simulink model "Model"  (R2016b)
settings: Solver=ode45  StartTime=0.0  StopTime=100  RelTol=1e-3
values from neighbouring files (symbols this model uses):
  b = 0.1    [main.m]
  g = 9.81    [main.m]
  H = [1 0 0 0 ... (first row only)    [main.m]
  K = lqr(A, B, Q, R )    [main.m]
  k = 0.15    [main.m]
  L = L_vec(i)    [main.m]
  M = 1    [main.m]
  m = 3/4    (= 0.75)    [main.m]
  Q = diag([1,1,1,1])    [main.m]
  R = 1    [main.m]
  theta_0 = 0    [main.m]
  theta_dot0 = 0    [main.m]
  x_0 = 0    [main.m]
  x_dot0 = 0    [main.m]
undefined symbols (not defined in the file or in its folder): delta, gamma, P_0, phi, X_0, y_0
libraries: simulink x3
settings Model: Creator=Erik  LastModifiedBy=sbuadu
settings DataIOCC: LimitDataPoints=on  SaveFormat=Array
settings OptimizationCC: BlockReduction=off  BooleanDataType=off  LifeSpan=inf
settings DebuggingCC: SaveWithParameterizedLinksMsg=none  UnderspecifiedInitializationDetection=Classic  MergeDetectMultiDrivingBlocksExec=none  SignalResolutionControl=TryResolveAllWithWarning  SFUnexpectedBacktrackingDiag=warning  SFNoUnconditionalDefaultTransitionDiag=warning  SFExecutionAtInitializationDiag=none
settings HardwareCC: ProdBitPerPointer=32  ProdBitPerSizeT=32  ProdBitPerPtrDiffT=32  ProdLargestAtomicFloat=None  ProdIntDivRoundTo=Undefined  ProdEndianess=Unspecified  ProdWordSize=32  ProdHWDeviceType=32-bit Generic  TargetUnknown=on
settings ModelReferenceCC: PropagateSignalLabelsOutOfModel=off
settings GRTTargetCC: TargetLangStandard=C89/C90 (ANSI)  GeneratePreprocessorConditionals=Disable all
settings ConfigComp: CovMetricSettings=dw  CovHtmlReporting=on  CovSaveCumulativeToWorkspaceVar=on  CovSaveSingleToWorkspaceVar=on  CovExternalEMLEnable=off  CovSFcnEnable=off

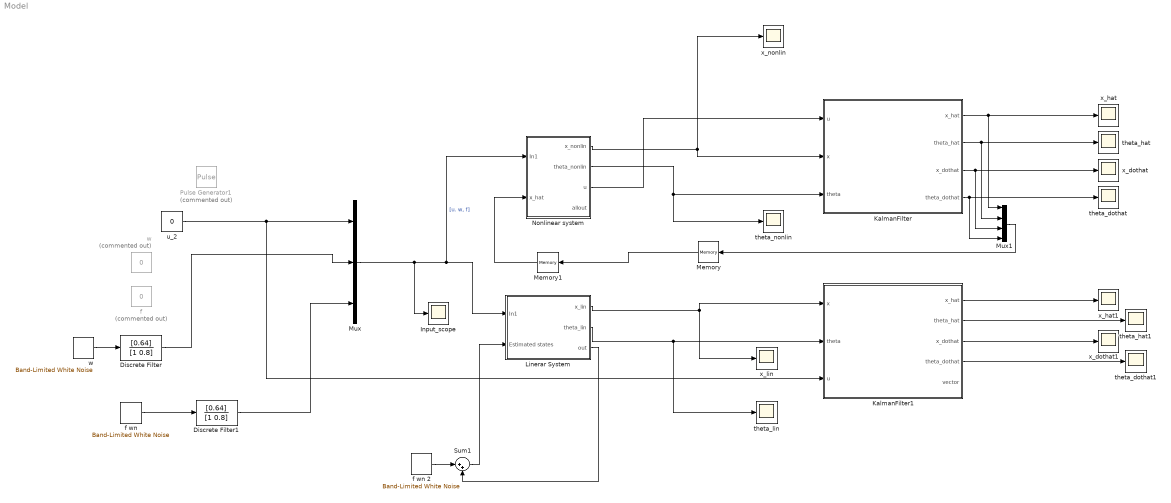
== system Model ==
  Discrete Filter : DiscreteFilter  Numerator=[0.64]  Denominator=[1 0.8]
  Discrete Filter1 : DiscreteFilter  Numerator=[0.64]  Denominator=[1 0.8]
  Input_scope : Scope
  KalmanFilter : Subsystem
  KalmanFilter1 : Subsystem
  Linerar System : Subsystem
  Memory : Memory  X0=X_0
  Memory1 : Memory  X0=X_0
  Mux : Mux  Inputs=3
  Mux1 : Mux
  "Nonlinear system " : Subsystem
  Pulse Generator1 : DiscretePulseGenerator  Commented=on  PulseType=Time based  Period=100  PhaseDelay=3
  Sum1 : Sum  Inputs=|++
  f : Constant  Commented=on  Value=0  SampleTime=0.01
  "f wn " : simulink/Sources/Band-Limited White Noise  Cov=10e-4  Ts=.001  seed=[23341]
  f wn 2 : simulink/Sources/Band-Limited White Noise  Cov=10e-7  Ts=.001  seed=[23341]
  theta_dothat : Scope
  theta_dothat1 : Scope
  theta_hat : Scope
  theta_hat1 : Scope
  theta_lin : Scope
  "theta_nonlin " : Scope
  u_2 : Constant  Value=0  SampleTime=0.01
  w : Constant  Commented=on  Value=0  SampleTime=0.01
  "w " : simulink/Sources/Band-Limited White Noise  Cov=10  Ts=.001  seed=[23341]
  x_dothat : Scope
  x_dothat1 : Scope
  x_hat : Scope
  x_hat1 : Scope
  x_lin : Scope
  x_nonlin : Scope
  wires:
  Mux/1 -> Input_scope/1, Linerar System/1(In1), "Nonlinear system "/1(In1)  "[u. w, f]"
  "Nonlinear system "/1(x_nonlin) -> KalmanFilter/2(x), x_nonlin/1
  "Nonlinear system "/2(theta_nonlin) -> KalmanFilter/3(theta), "theta_nonlin "/1
  u_2/1 -> KalmanFilter1/3("u "), Mux/1
  Linerar System/1(x_lin) -> KalmanFilter1/1(x), x_lin/1
  Linerar System/2(theta_lin) -> theta_lin/1, KalmanFilter1/2(theta)
  KalmanFilter/1(x_hat) -> Mux1/1, x_hat/1
  KalmanFilter/2(theta_hat) -> Mux1/2, theta_hat/1
  KalmanFilter/4(theta_dothat) -> Mux1/4, theta_dothat/1
  KalmanFilter1/1(x_hat) -> x_hat1/1
  KalmanFilter1/2(theta_hat) -> theta_hat1/1
  KalmanFilter1/3(x_dothat) -> x_dothat1/1
  KalmanFilter1/4(theta_dothat) -> theta_dothat1/1
  Mux1/1 -> Memory/1
  KalmanFilter/3(x_dothat) -> Mux1/3, x_dothat/1
  "Nonlinear system "/3(u) -> KalmanFilter/1("u ")
  Memory/1 -> Memory1/1
  Discrete Filter1/1 -> Mux/3
  "w "/1 -> Discrete Filter/1
  "f wn "/1 -> Discrete Filter1/1
  Discrete Filter/1 -> Mux/2
  Memory1/1 -> "Nonlinear system "/2(x_hat)
  Sum1/1 -> Linerar System/2(Estimated states)
  f wn 2/1 -> Sum1/1
  Linerar System/3("out ") -> Sum1/2

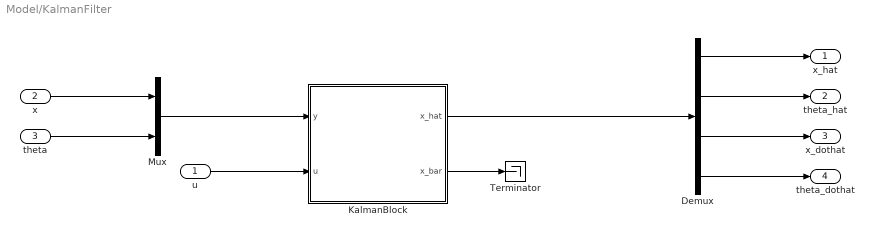
== system Model/KalmanFilter ==
  "u " : Inport
  x : Inport  Port=2
  theta : Inport  Port=3
  Demux : Demux
  KalmanBlock : Subsystem
  Mux : Mux  Inputs=2
  Terminator : Terminator
  x_hat : Outport
  theta_hat : Outport  Port=2
  x_dothat : Outport  Port=3
  theta_dothat : Outport  Port=4
  wires:
  Mux/1 -> KalmanBlock/1("y ")
  "u "/1 -> KalmanBlock/2("u ")
  x/1 -> Mux/1
  theta/1 -> Mux/2
  KalmanBlock/1(x_hat) -> Demux/1
  Demux/1 -> x_hat/1
  Demux/2 -> theta_hat/1
  Demux/3 -> x_dothat/1
  Demux/4 -> theta_dothat/1
  KalmanBlock/2(x_bar) -> Terminator/1

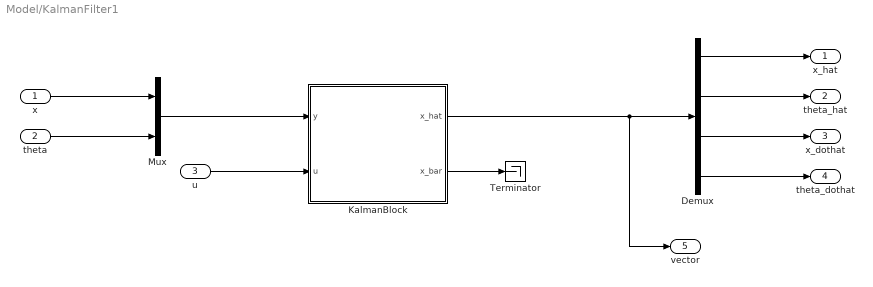
== system Model/KalmanFilter1 ==
  x : Inport
  theta : Inport  Port=2
  "u " : Inport  Port=3
  Demux : Demux
  KalmanBlock : Subsystem
  Mux : Mux  Inputs=2
  Terminator : Terminator
  x_hat : Outport
  theta_hat : Outport  Port=2
  x_dothat : Outport  Port=3
  theta_dothat : Outport  Port=4
  vector : Outport  Port=5
  wires:
  Mux/1 -> KalmanBlock/1("y ")
  "u "/1 -> KalmanBlock/2("u ")
  x/1 -> Mux/1
  theta/1 -> Mux/2
  KalmanBlock/1(x_hat) -> vector/1, Demux/1
  Demux/1 -> x_hat/1
  Demux/2 -> theta_hat/1
  Demux/3 -> x_dothat/1
  Demux/4 -> theta_dothat/1
  KalmanBlock/2(x_bar) -> Terminator/1

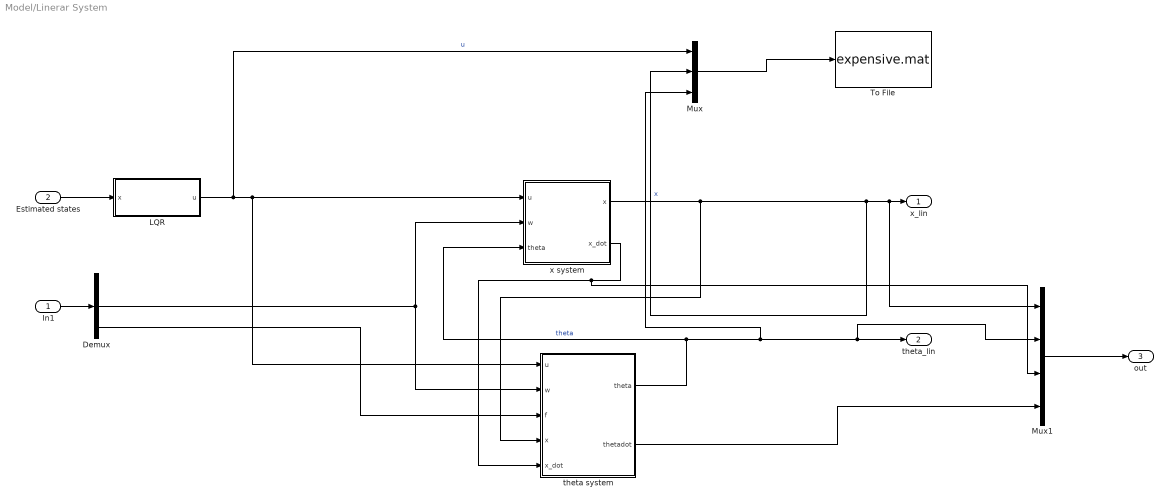
== system Model/Linerar System ==
  In1 : Inport
  Estimated states : Inport  Port=2
  Demux : Demux  Outputs=3
  LQR : Subsystem
  Mux : Mux  Inputs=3
  Mux1 : Mux
  To File : ToFile  Filename=expensive.mat  MatrixName=data
  "theta system " : Subsystem
  x system : Subsystem
  x_lin : Outport
  theta_lin : Outport  Port=2
  "out " : Outport  Port=3
  wires:
  Demux/2 -> "theta system "/2(w), x system/2(w)
  Demux/3 -> "theta system "/3(f)
  x system/2(x_dot) -> Mux1/3, "theta system "/5(x_dot)
  In1/1 -> Demux/1
  Estimated states/1 -> LQR/1(x)
  LQR/1(u) -> Mux/1, "theta system "/1("u "), x system/1("u ")  "u"
  x system/1(x) -> "theta system "/4(x), Mux/2, Mux1/1, x_lin/1  "x"
  "theta system "/1(theta) -> Mux/3, Mux1/2, theta_lin/1, x system/3(theta)  "theta"
  Mux/1 -> To File/1
  "theta system "/2("thetadot ") -> Mux1/4
  Mux1/1 -> "out "/1

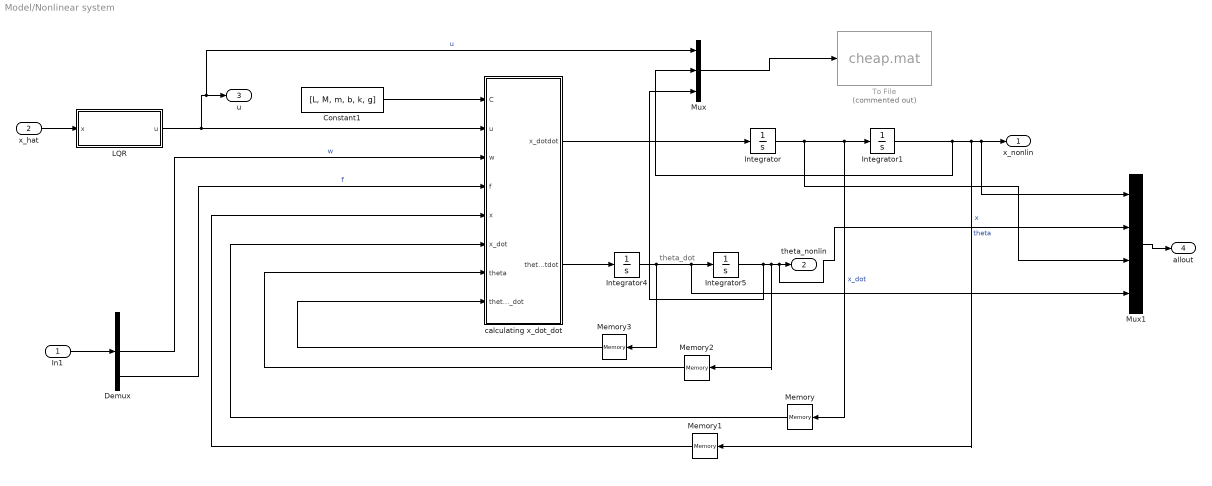
== system Model/Nonlinear system  ==
  note: theta_dot
  In1 : Inport
  x_hat : Inport  Port=2
  Constant1 : Constant  Value=[L, M, m, b, k, g]  SampleTime=0.01
  Demux : Demux  Outputs=3
  Integrator{,1,4..5} (4 alike) : Integrator
  LQR : Subsystem
  Memory : Memory  X0=x_dot0
  Memory1 : Memory  X0=x_0
  Memory2 : Memory  X0=theta_0
  Memory3 : Memory  X0=theta_dot0
  Mux : Mux  Inputs=3
  Mux1 : Mux
  To File : ToFile  Commented=on  Filename=cheap.mat  MatrixName=data
  calculating x_dot_dot : MATLAB Function  TreatAsAtomicUnit=on
  x_nonlin : Outport
  theta_nonlin : Outport  Port=2
  u : Outport  Port=3
  "allout " : Outport  Port=4
  wires:
  In1/1 -> Demux/1
  LQR/1(u) -> Mux/1, u/1, calculating x_dot_dot/2(u)  "u"
  Demux/2 -> calculating x_dot_dot/3(w)  "w"
  Demux/3 -> calculating x_dot_dot/4(f)  "f"
  calculating x_dot_dot/1(x_dotdot) -> Integrator/1
  Integrator/1 -> Mux1/3, Memory/1, Integrator1/1  "x_dot"
  Integrator1/1 -> Mux/2, Memory1/1, Mux1/1, x_nonlin/1  "x"
  Constant1/1 -> calculating x_dot_dot/1(C)
  calculating x_dot_dot/2(theta_dotdot) -> Integrator4/1
  Integrator4/1 -> Memory3/1, Mux1/4, Integrator5/1
  Integrator5/1 -> Mux/3, Memory2/1, Mux1/2, theta_nonlin/1  "theta"
  Memory1/1 -> calculating x_dot_dot/5(x)
  Memory/1 -> calculating x_dot_dot/6(x_dot)
  Memory2/1 -> calculating x_dot_dot/7(theta)
  Memory3/1 -> calculating x_dot_dot/8(theta_dot)
  x_hat/1 -> LQR/1(x)
  Mux/1 -> To File/1
  Mux1/1 -> "allout "/1

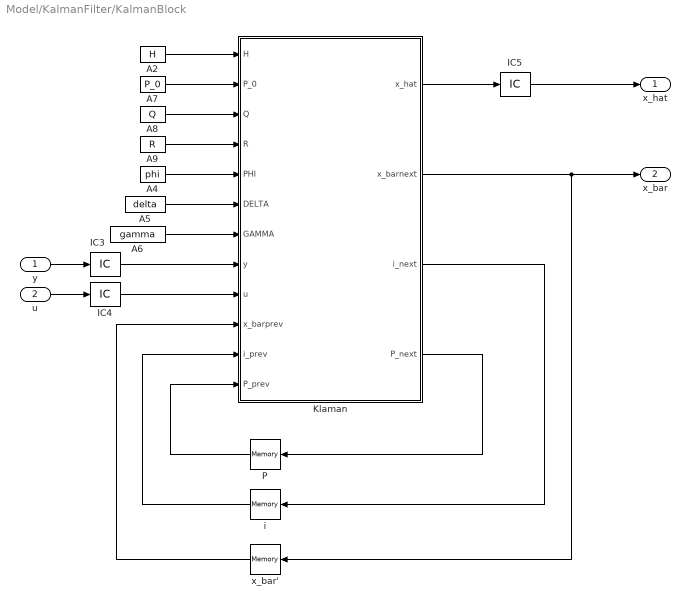
== system Model/KalmanFilter/KalmanBlock ==
  "y " : Inport
  "u " : Inport  Port=2
  A2 : Constant  Value=H
  A4 : Constant  Value=phi
  A5 : Constant  Value=delta
  A6 : Constant  Value=gamma
  A7 : Constant  Value=P_0
  A8 : Constant  Value=Q
  A9 : Constant  Value=R
  IC3 : InitialCondition  Value=y_0
  IC4 : InitialCondition  Value=0
  IC5 : InitialCondition  Value=X_0
  Klaman : MATLAB Function  TreatAsAtomicUnit=on
  P : Memory  X0=P_0
  "i " : Memory
  x_bar' : Memory  X0=X_0
  x_hat : Outport
  x_bar : Outport  Port=2
  wires:
  A8/1 -> Klaman/3(Q)
  A6/1 -> Klaman/7(GAMMA)
  A4/1 -> Klaman/5(PHI)
  Klaman/2(x_barnext) -> x_bar'/1, x_bar/1
  Klaman/3(i_next) -> "i "/1
  Klaman/1(x_hat) -> IC5/1
  Klaman/4(P_next) -> P/1
  A2/1 -> Klaman/1(H)
  A5/1 -> Klaman/6(DELTA)
  IC4/1 -> Klaman/9(u)
  A7/1 -> Klaman/2(P_0)
  "u "/1 -> IC4/1
  A9/1 -> Klaman/4(R)
  "y "/1 -> IC3/1
  IC5/1 -> x_hat/1
  IC3/1 -> Klaman/8(y)
  "i "/1 -> Klaman/11(i_prev)
  P/1 -> Klaman/12(P_prev)
  x_bar'/1 -> Klaman/10(x_barprev)

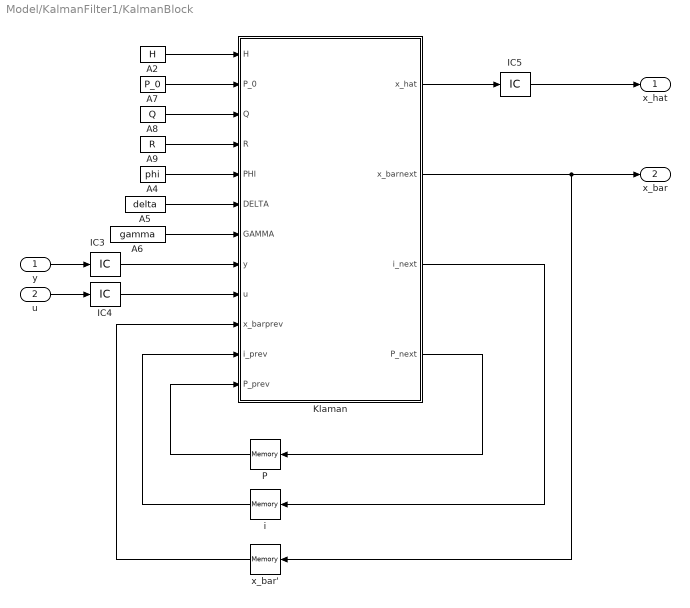
== system Model/KalmanFilter1/KalmanBlock ==
  "y " : Inport
  "u " : Inport  Port=2
  A2 : Constant  Value=H
  A4 : Constant  Value=phi
  A5 : Constant  Value=delta
  A6 : Constant  Value=gamma
  A7 : Constant  Value=P_0
  A8 : Constant  Value=Q
  A9 : Constant  Value=R
  IC3 : InitialCondition  Value=y_0
  IC4 : InitialCondition  Value=0
  IC5 : InitialCondition  Value=X_0
  Klaman : MATLAB Function  TreatAsAtomicUnit=on
  P : Memory  X0=P_0
  "i " : Memory
  x_bar' : Memory  X0=X_0
  x_hat : Outport
  x_bar : Outport  Port=2
  wires:
  A8/1 -> Klaman/3(Q)
  A6/1 -> Klaman/7(GAMMA)
  A4/1 -> Klaman/5(PHI)
  Klaman/2(x_barnext) -> x_bar'/1, x_bar/1
  Klaman/3(i_next) -> "i "/1
  Klaman/1(x_hat) -> IC5/1
  Klaman/4(P_next) -> P/1
  A2/1 -> Klaman/1(H)
  A5/1 -> Klaman/6(DELTA)
  IC4/1 -> Klaman/9(u)
  A7/1 -> Klaman/2(P_0)
  "u "/1 -> IC4/1
  A9/1 -> Klaman/4(R)
  "y "/1 -> IC3/1
  IC5/1 -> x_hat/1
  IC3/1 -> Klaman/8(y)
  "i "/1 -> Klaman/11(i_prev)
  P/1 -> Klaman/12(P_prev)
  x_bar'/1 -> Klaman/10(x_barprev)

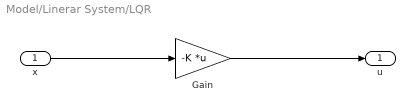
== system Model/Linerar System/LQR ==
  x : Inport
  Gain : Gain  Gain=-K  Multiplication=Matrix(K*u)
  u : Outport
  wires:
  Gain/1 -> u/1
  x/1 -> Gain/1

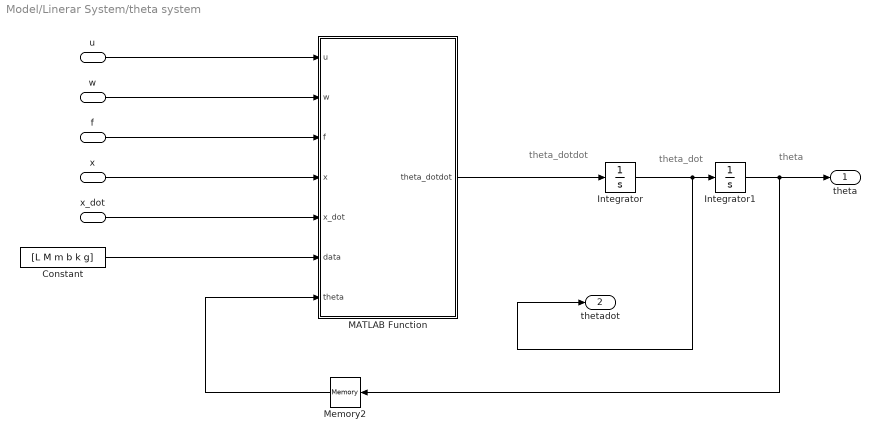
== system Model/Linerar System/theta system  ==
  note: theta
  note: theta_dotdot
  note: theta_dot
  "u " : Inport
  w : Inport  Port=2
  f : Inport  Port=3
  x : Inport  Port=4
  x_dot : Inport  Port=5
  Constant : Constant  Value=[L M m b k g]  VectorParams1D=off  SampleTime=0.01
  Integrator : Integrator
  Integrator1 : Integrator
  MATLAB Function : MATLAB Function  TreatAsAtomicUnit=on
  Memory2 : Memory  X0=theta_0
  theta : Outport
  "thetadot " : Outport  Port=2
  wires:
  MATLAB Function/1(theta_dotdot) -> Integrator/1
  Integrator/1 -> "thetadot "/1, Integrator1/1
  "u "/1 -> MATLAB Function/1(u)
  w/1 -> MATLAB Function/2(w)
  x/1 -> MATLAB Function/4(x)
  Integrator1/1 -> Memory2/1, theta/1
  Constant/1 -> MATLAB Function/6(data)
  f/1 -> MATLAB Function/3(f)
  x_dot/1 -> MATLAB Function/5(x_dot)
  Memory2/1 -> MATLAB Function/7(theta)

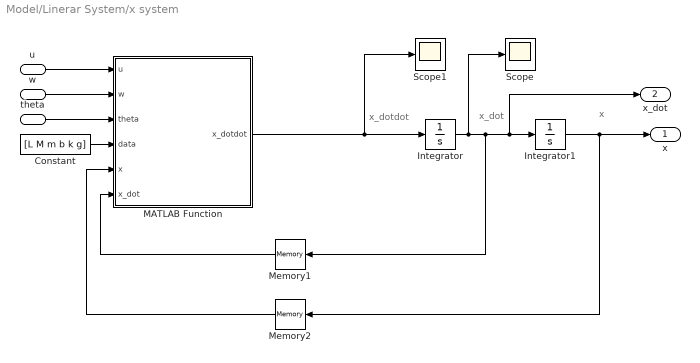
== system Model/Linerar System/x system ==
  note: x
  note: x_dotdot
  note: x_dot
  "u " : Inport
  w : Inport  Port=2
  theta : Inport  Port=3
  Constant : Constant  Value=[L M m b k g]  VectorParams1D=off  SampleTime=0.01
  Integrator : Integrator
  Integrator1 : Integrator
  MATLAB Function : MATLAB Function  TreatAsAtomicUnit=on
  Memory1 : Memory  X0=x_dot0
  Memory2 : Memory  X0=x_0
  Scope : Scope
  Scope1 : Scope
  x : Outport
  x_dot : Outport  Port=2
  wires:
  Memory1/1 -> MATLAB Function/6(x_dot)
  "u "/1 -> MATLAB Function/1(u)
  w/1 -> MATLAB Function/2(w)
  theta/1 -> MATLAB Function/3(theta)
  Integrator1/1 -> Memory2/1, x/1
  Memory2/1 -> MATLAB Function/5(x)
  Constant/1 -> MATLAB Function/4(data)
  Integrator/1 -> Scope/1, Integrator1/1, x_dot/1, Memory1/1
  MATLAB Function/1(x_dotdot) -> Scope1/1, Integrator/1

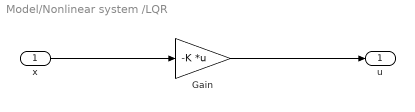
== system Model/Nonlinear system /LQR ==
  x : Inport
  Gain : Gain  Gain=-K  Multiplication=Matrix(K*u)
  u : Outport
  wires:
  Gain/1 -> u/1
  x/1 -> Gain/1

== matlab function Model/Linerar System/x system/MATLAB Function ==
  data: u input; w input; theta input; data input; x_dotdot output; x input; x_dot input
function x_dotdot  = fcn(u, w, theta, data, x, x_dot)
L = data(1);
M = data(2);
m = data(3);
b = data(4);
k = data(5);
g = data(6);

% theta = theta * 180 / pi;

x_dotdot=(u - w - m * g * theta - b * x_dot - k * x) / M;


end

== matlab function Model/KalmanFilter/KalmanBlock/Klaman ==
  data: H input; P_0 input; Q input; R input; PHI input; DELTA input; GAMMA input; y input; u input; x_barprev input; i_prev input; P_prev input; x_hat output; x_barnext output; i_next output; P_next output
function [x_hat,x_barnext,i_next,P_next] = KalmanFilter(H,P_0,Q,R,PHI,DELTA,GAMMA,y,u,x_barprev,i_prev,P_prev)
I=eye(4);
if i_prev ==0
    x_barnext=x_barprev;
    x_hat=x_barprev;
    P_next=P_0;
else
    K=P_prev*(H')*inv(H*P_prev*(H')+R);
    x_hat=x_barprev+K*(y-H*x_barprev);
    P_hat=(I-K*H)*P_prev*(I-K*H)'+K*R*K';
    
    x_barnext=PHI*x_hat+DELTA*u;
    P_next=PHI*P_hat*PHI'+GAMMA*Q*GAMMA';
end

i_next=i_prev+1;
end

== matlab function Model/Linerar System/theta system /MATLAB Function ==
  data: u input; w input; f input; x input; x_dot input; data input; theta input; theta_dotdot output
function theta_dotdot  = fcn(u, w, f, x, x_dot, data, theta)
L = data(1);
M = data(2);
m = data(3);
b = data(4);
k = data(5);
g = data(6);

% theta = theta * 180 / pi;

theta_dotdot=(-u + w + (m + M) * g * theta - (M / m) * f + b * x_dot + k * x)/(L * M);

end

== matlab function Model/Nonlinear system /calculating x_dot_dot ==
  data: C input; u input; x_dotdot output; w input; f input; x input; x_dot input; theta input; theta_dot input; theta_dotdot output
function [x_dotdot, theta_dotdot]= fcn(C,u, w, f, x, x_dot, theta, theta_dot)
%extracting the know parameters from vector C
L = C(1); 
M= C(2); 
m=C(3); 
b = C(4); 
k = C(5); 
g = C(6);

%calculating x_dot_dot
 x_dotdot = (u - f - w + f*cos(theta)^2 ...
            + m*L*theta_dot^2*sin(theta) ...
            -m*g*sin(theta)*cos(theta)...
            -b*x_dot -k*x )/(M + m*sin(theta)^2); 

%calculating theta_dot_dot
 theta_dotdot = (-u*cos(theta)+w*cos(theta)...
                   -M*L*theta_dot^2*sin(theta)*cos(theta)...
                    +(m+M)*g*sin(theta)-(M/m)*f*cos(theta)...
                    +b*x_dot*cos(theta)...
                    + k*x*cos(theta))/(L*(M+m*sin(theta)^2));

== matlab function Model/KalmanFilter1/KalmanBlock/Klaman ==
  data: H input; P_0 input; Q input; R input; PHI input; DELTA input; GAMMA input; y input; u input; x_barprev input; i_prev input; P_prev input; x_hat output; x_barnext output; i_next output; P_next output
function [x_hat, x_barnext, i_next, P_next] = KalmanFilter(H, P_0, Q, R, PHI, DELTA, GAMMA, y, u, x_barprev, i_prev, P_prev)
I = eye(4);
if i_prev == 0
    x_barnext = x_barprev;
    x_hat = x_barprev;
    P_next = P_0;
else
    K = P_prev * (H') * inv(H * P_prev * (H') + R);
    x_hat = x_barprev + K * (y - H * x_barprev);
    P_hat = (I - K * H) * P_prev * (I - K * H)' + K * R * K';
    
    x_barnext = PHI * x_hat + DELTA * u;
    P_next = PHI * P_hat * PHI' + GAMMA * Q * GAMMA';
end

i_next=i_prev+1;
end
